simulink model "blackbox_diagram_deneme1_togi"  (R2023b)
settings: Solver=VariableStepAuto  StartTime=0.0  StopTime=10.0  RelTol=1e-3
PreLoadFcn:
  | addpath(genpath('lib'))
InitFcn:
  | addpath('lib')
model workspace (MAT data in the model file):
  distance = Simulink.LookupTable
  distance.Table = Simulink.lookuptable.Table
  distance.Table.Value = [1 2]
  distance.Table.Dimensions = [1 2]
  distance.Table.DataType = 'auto'
  distance.Table.FieldName = 'Table'
  distance.Breakpoints = Simulink.lookuptable.Breakpoint
  distance.Breakpoints.Value = [1 2]
  distance.Breakpoints.TunableSizeName = 'N1'
  distance.Breakpoints.Dimensions = [1 2]
  distance.Breakpoints.DataType = 'auto'
  distance.Breakpoints.FieldName = 'BP1'
  distance.AllowMultipleInstancesOfTypeToHaveDifferentTableBreakpointSizes = 0
  distance.SupportTunableSize = 0
  distance.StructTypeInfo = Simulink.lookuptable.StructTypeInfo
  distance.StructTypeInfo.DataScope = 'Auto'
  frequency = Simulink.LookupTable
  frequency.Table = Simulink.lookuptable.Table
  frequency.Table.Value = [1 2]
  frequency.Table.Dimensions = [1 2]
  frequency.Table.DataType = 'auto'
  frequency.Table.FieldName = 'Table'
  frequency.Breakpoints = Simulink.lookuptable.Breakpoint
  frequency.Breakpoints.Value = [1 2]
  frequency.Breakpoints.TunableSizeName = 'N1'
  frequency.Breakpoints.Dimensions = [1 2]
  frequency.Breakpoints.DataType = 'auto'
  frequency.Breakpoints.FieldName = 'BP1'
  frequency.AllowMultipleInstancesOfTypeToHaveDifferentTableBreakpointSizes = 0
  frequency.SupportTunableSize = 0
  frequency.StructTypeInfo = Simulink.lookuptable.StructTypeInfo
  frequency.StructTypeInfo.DataScope = 'Auto'
libraries: commrflib2 x1
settings Model: Creator=Tolga-Evry  LastModifiedBy=Tolga-Evry

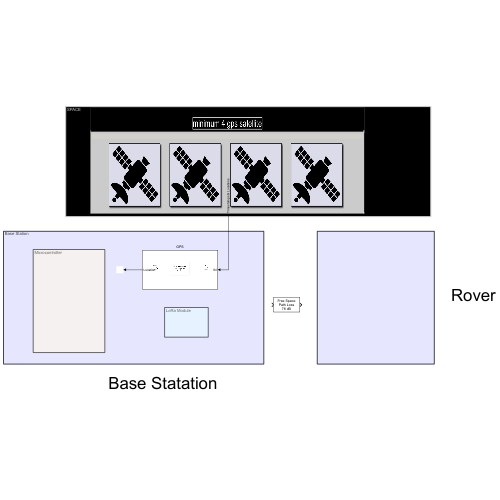
[thumbnail: Simulink's stored preview of the top-level diagram]
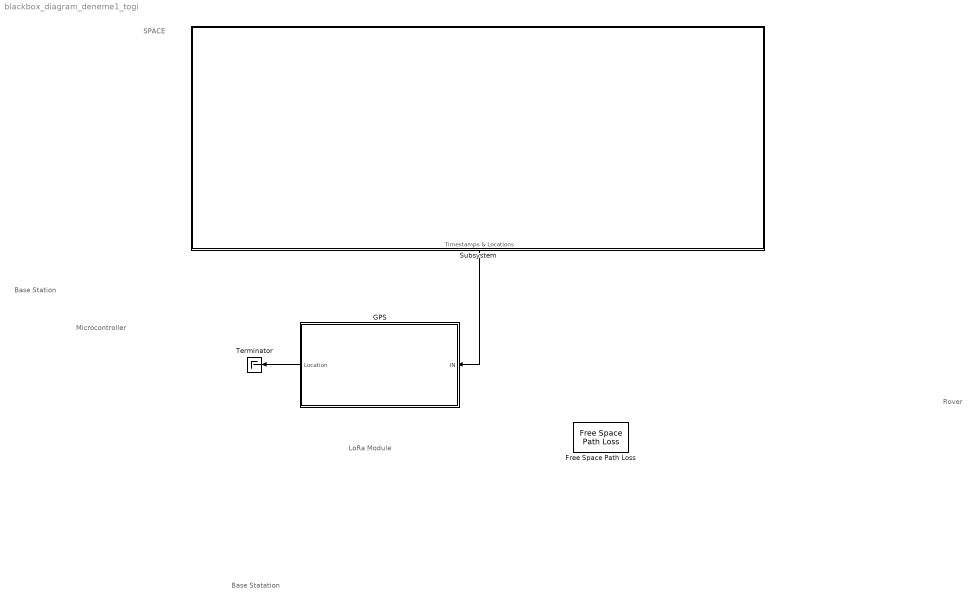
== system blackbox_diagram_deneme1_togi ==
  note: Base Statation
  note: Base Station
  note: Rover
  note: Microcontroller
  note: LoRa Module
  note: SPACE
  Free Space Path Loss : commrflib2/Free Space Path Loss  mode=Distance and Frequency  dB=10  d=0.100  fc=1920
  GPS : Subsystem
      mask Display: image('GPS_internal_structer_2.png');
  Subsystem : Subsystem
      settings: PortSchema="{\"entries\":[{\"content\":{\"sides\":[{\"content\":{},\"type\":\"ConnectorPlacement.EquallySpacedRectSide\",\"uuid\":\"4e20a065-8941-4c55-b103-51b4c542c2bd\"},{\"content\":{\"side\":\"RIGHT\"},\"type\":\"ConnectorPlacement.EquallySpacedRectSide\",\"uuid\":\"e0e67d93-da9d-46f5-a60e-8146c03d855c\"},{\"content\":{\"side\":\"TOP\"},\"type\":\"ConnectorPlacement.EquallySpacedRectSide\",\"uuid\":\"5a84b0c8-526c-42be-b803-23b85f884774\"},{\"content\":{\"connectorIds\":[\"Out1\"],\"side\":\"BOTTOM\"},\"type\":\"ConnectorPlacement.EquallySpacedRectSide\",\"uuid\":\"f9781b0a-2a89-4dc8-b07e-b33ac5e0f8fd\"}]},\"type\":\"ConnectorPlacement.EquallySpacedConnector\",\"uuid\":\"cff0439c-cb45-4810-be78-65312b977715\"}],\"packageUris\":[\"http://schema.mathworks.com/mf0/Connector/R2020b\"],\"version\":\"1.0\"}"
      mask Display: image('gps_satellites.png');
  Terminator : Terminator
  wires:
  Subsystem/1(Timestamps & Locations) -> GPS/1(IN)
  GPS/1(Location) -> Terminator/1

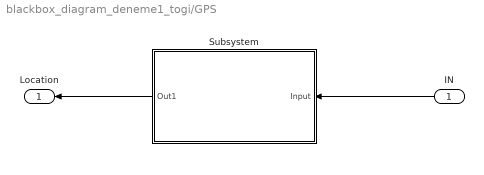
== system blackbox_diagram_deneme1_togi/GPS ==
  IN : Inport
  Subsystem : Subsystem
      mask Display: fprintf('Location Estimation using \n timestamp datas from \n satellite');
  Location : Outport
  wires:
  IN/1 -> Subsystem/1(Input)
  Subsystem/1(Out1) -> Location/1

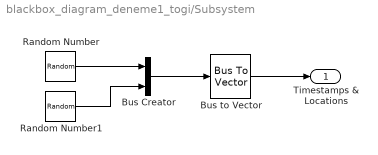
== system blackbox_diagram_deneme1_togi/Subsystem ==
  Bus Creator : BusCreator  Inputs=2
  Bus to Vector : BusToVector
  Random Number : RandomNumber  SampleTime=0.1
  Random Number1 : RandomNumber  SampleTime=0.1
  Timestamps & Locations : Outport
  wires:
  Bus Creator/1 -> Bus to Vector/1
  Bus to Vector/1 -> Timestamps & Locations/1
  Random Number/1 -> Bus Creator/1
  Random Number1/1 -> Bus Creator/2

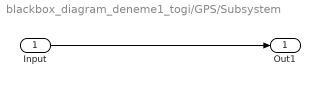
== system blackbox_diagram_deneme1_togi/GPS/Subsystem ==
  Input : Inport
  Out1 : Outport
  wires:
  Input/1 -> Out1/1
